simulink model "CT_T1_nivel"  (Simulink 7.0)
settings: Solver=ode45  StartTime=0.0  StopTime=120  FixedStep=Tsamp  RelTol=1e-5
settings Model: Creator=Administrator  LastModifiedBy=Equipo-Servo
settings SolverCC: MaxConsecutiveMinStep=10
settings DebuggingCC: SaveWithParameterizedLinksMsg=none  SignalResolutionControl=TryResolveAllWithWarning  MultiTaskDSMMsg=warning  MultiTaskCondExecSysMsg=none  StrictBusMsg=None
settings RTWCC: ProcessScript=grt_make_rtw_hook  IncludeERTFirstTime=on
settings CodeAppCC: CustomSymbolStrType=$N$R$M_T
settings GRTTargetCC: TargetFcnLib=ansi_tfl_tmw.mat

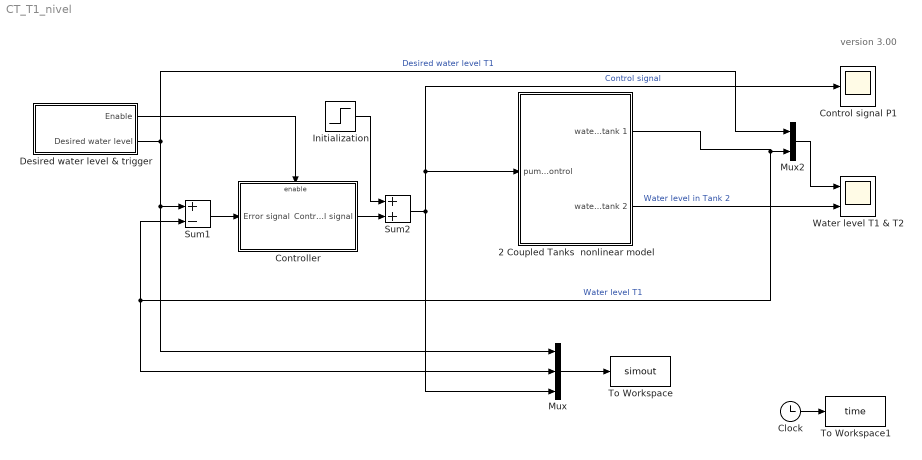
== system CT_T1_nivel ==
  note: version 3.00
  2 Coupled Tanks  nonlinear model : Subsystem  mask{A=0.01389, eta=2.2e-3, a1=50.265e-6, a2=50.265e-6}
      mask prompts: A "Cross-sectional area of the tanks"; eta "Constant relating the control voltage witch the water flow from the pump"; a1 "Tank 1 outlet area"; a2 "Tank 2 outlet area"
      mask Display: disp('Tanks')
  Clock : Clock
  Control signal P1 : Scope
      settings: TimeRange=600  YMin=0  MaxDataPoints=500000
  Controller : Subsystem
      mask Display: disp('Controller')
  Desired water level & trigger : Subsystem
  Initialization : Step  Time=35  Before=5  After=2.7  SampleTime=0
  Mux : Mux  Inputs=3
  Mux2 : Mux  Inputs=2
  Sum1 : Sum  Inputs=+-  SaturateOnIntegerOverflow=on  InputSameDT=on
  Sum2 : Sum  SaturateOnIntegerOverflow=on  InputSameDT=on
  To Workspace : ToWorkspace  VariableName=simout  SampleTime=0.1  SaveFormat=Structure With Time
  To Workspace1 : ToWorkspace  VariableName=time  SampleTime=0.1
  Water level T1 & T2 : Scope  NumInputPorts=2
      settings: TimeRange=600  YMin=0~0  YMax=30~30  MaxDataPoints=500000
  wires:
  Clock/1 -> To Workspace1/1
  2 Coupled Tanks  nonlinear model/1(water level in tank 1) -> Mux2/2, Sum1/2, Mux/2  "Water level T1"
  2 Coupled Tanks  nonlinear model/2(water level in tank 2) -> Water level T1 & T2/2  "Water level in Tank 2"
  Mux/1 -> To Workspace/1
  Mux2/1 -> Water level T1 & T2/1
  Desired water level & trigger/2(Desired water level) -> Mux2/1, Sum1/1, Mux/1  "Desired water level T1"
  Sum1/1 -> Controller/1(Error signal)
  Controller/1(Control signal) -> Sum2/2
  Initialization/1 -> Sum2/1
  Desired water level & trigger/1(Enable) -> Controller/Enable
  Sum2/1 -> Control signal P1/1, 2 Coupled Tanks  nonlinear model/1(pump control), Mux/3  "Control signal"

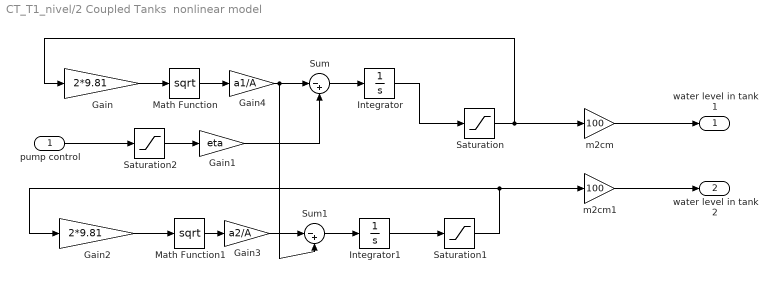
== system CT_T1_nivel/2 Coupled Tanks  nonlinear model ==
  pump control : Inport
  Gain : Gain  Gain=2*9.81
  Gain1 : Gain  Gain=eta
  Gain2 : Gain  Gain=2*9.81
  Gain3 : Gain  Gain=a2/A
  Gain4 : Gain  Gain=a1/A
  Integrator : Integrator
  Integrator1 : Integrator
  Math Function : Math  Operator=sqrt  SaturateOnIntegerOverflow=on
  Math Function1 : Math  Operator=sqrt  SaturateOnIntegerOverflow=on
  Saturation : Saturate  UpperLimit=0.3  LowerLimit=0
  Saturation1 : Saturate  UpperLimit=0.3  LowerLimit=0
  Saturation2 : Saturate  UpperLimit=5  LowerLimit=0
  Sum : Sum  Inputs=|-+
  Sum1 : Sum  Inputs=|-+
  m2cm : Gain  Gain=100
  m2cm1 : Gain  Gain=100
  water level in tank 1 : Outport
  water level in tank 2 : Outport  Port=2
  wires:
  Saturation1/1 -> Gain2/1, m2cm1/1
  Saturation2/1 -> Gain1/1
  Saturation/1 -> Gain/1, m2cm/1
  Gain4/1 -> Sum/1, Sum1/2
  Gain1/1 -> Sum/2
  pump control/1 -> Saturation2/1
  Gain3/1 -> Sum1/1
  Sum1/1 -> Integrator1/1
  Math Function1/1 -> Gain3/1
  Gain2/1 -> Math Function1/1
  Integrator1/1 -> Saturation1/1
  Sum/1 -> Integrator/1
  Math Function/1 -> Gain4/1
  Gain/1 -> Math Function/1
  Integrator/1 -> Saturation/1
  m2cm/1 -> water level in tank 1/1
  m2cm1/1 -> water level in tank 2/1

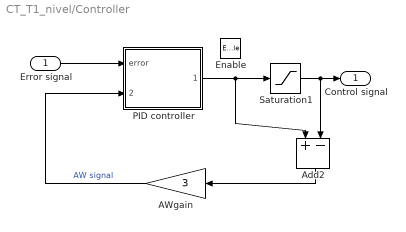
== system CT_T1_nivel/Controller ==
  Error signal : Inport
  Enable : EnablePort
  AWgain : Gain  Orientation=left  Gain=3
  Add2 : Sum  Orientation=down  Inputs=+-
  PID controller : Subsystem
      mask Display: disp('PID')
  Saturation1 : Saturate  UpperLimit=2.3  LowerLimit=-2.7
  Control signal : Outport
  wires:
  AWgain/1 -> PID controller/2(anti-windup signal)  "AW signal"
  Add2/1 -> AWgain/1
  PID controller/1(control signal) -> Saturation1/1, Add2/1
  Saturation1/1 -> Add2/2, Control signal/1
  Error signal/1 -> PID controller/1(error)

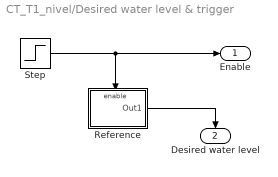
== system CT_T1_nivel/Desired water level & trigger ==
  Reference : Subsystem
  Step : Step  Time=35  SampleTime=0
  Enable : Outport
  Desired water level : Outport  Orientation=down  Port=2
  wires:
  Step/1 -> Reference/Enable, Enable/1
  Reference/1(Out1) -> Desired water level/1

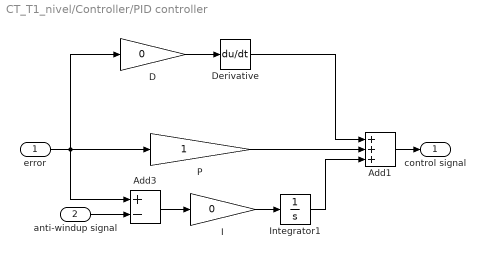
== system CT_T1_nivel/Controller/PID controller ==
  error : Inport
  anti-windup signal : Inport  Port=2
  Add1 : Sum  Inputs=+++
  Add3 : Sum  Inputs=+-
  D : Gain  Gain=0
  Derivative : Derivative
  I : Gain  Gain=0
  Integrator1 : Integrator
  P : Gain
  control signal : Outport
  wires:
  error/1 -> P/1, Add3/1, D/1
  I/1 -> Integrator1/1
  Add3/1 -> I/1
  Add1/1 -> control signal/1
  anti-windup signal/1 -> Add3/2
  D/1 -> Derivative/1
  Derivative/1 -> Add1/1
  P/1 -> Add1/2
  Integrator1/1 -> Add1/3

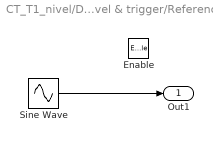
== system CT_T1_nivel/Desired water level & trigger/Reference ==
  Enable : EnablePort
  Sine Wave : Sin  Amplitude=3  Bias=20  Frequency=2*pi*0.01  Phase=-3.66  SampleTime=0
  Out1 : Outport
  wires:
  Sine Wave/1 -> Out1/1
